simulink model "nmc_full_body_simmechanics_3fbl_2014a"  (R2014a)
settings: Solver=ode23s  StartTime=0.0  StopTime=40  FixedStep=1e-3  MaxStep=ts_max  RelTol=1e-3  AbsTol=1e-4
InitFcn:
  | addpath('../lib');
  | addpath('./init_script');
  | nms_model_MechInit
  | nms_model_ControlInit
undefined symbols (not defined in the file): alphaFmGas, alphaFmGlu, alphaFmHam, alphaFmSol, alphaFmVas, alphaLceHam, alphaLceHfl, alphaLceTa, alphaLceTa1, Amp, amp_var, D12_F, D12_S, D12_T, D13_F, D1G_F, D1G_HAT, D1G_S, D1G_T, freq, freq_var, In_F, In_HAT, In_S, In_T, k_gx, k_gy, k_pressure, m_F, m_HAT, m_S, m_T, mu_slide, mu_stick, sgn, ThPos, v_gx_max, v_gy_max, v_max_pressure, vLimit
libraries: mblibv1 x60, simulink x30, simulink_extras x4, nmc x4
(part 2 of 3)

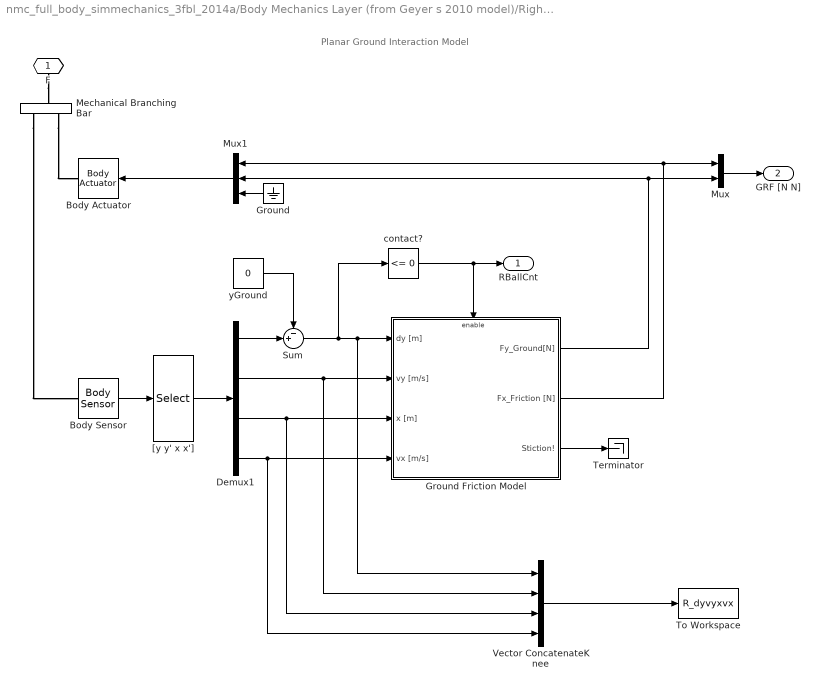
== system nmc_full_body_simmechanics_3fbl_2014a/Body Mechanics Layer (from Geyer s 2010 model)/Right Ball Contact ==
  note: Planar Ground Interaction Model
  Body Actuator : mblibv1/Sensors &  Actuators/Body Actuator  UpdateFromCAD=off  PhysicalDomain=Mechanical  PortType=blob  ActuationStyle=Force  AngleUnits=deg  ArcVelocityUnits=deg/s  ArcAccelerationUnits=deg/s^2  CoordPositionUnits=m  VelocityUnits=m/s  AccelerationUnits=m/s^2  ForceUnits=N  TorqueUnits=N-m  ActiveIO=on  Width=3  DialogClass=MechanicalActuatorBlock  ReferenceFrame=Absolute (World)  Angle=off  CoordPosition=on  Force=on  Torque=off
  Body Sensor : mblibv1/Sensors &  Actuators/Body Sensor  UpdateFromCAD=off  PhysicalDomain=Mechanical  PortType=blob  Muxed=on  Pose=off  Angle=on  AngleUnits=deg  ArcVelocity=off  ArcVelocityUnits=deg/s  ArcAcceleration=off  ArcAccelerationUnits=deg/s^2  CoordPosition=on  CoordPositionUnits=m  Velocity=on  VelocityUnits=m/s  Acceleration=off  AccelerationUnits=m/s^2  Quaternion=on  QuaternionDT=off  QuaternionDDT=off  QuaternionUnits=off  OutputVector=[ 3 3 ]  ActiveIO=on  Width=6  DialogClass=MechanicalSensorBlock  ReferenceFrame=Absolute (World)
  Demux1 : Demux
  Ground : Ground
  Ground Friction Model : Subsystem
  Mechanical Branching Bar : mblibv1/Utilities/Mechanical Branching Bar  LConnTagsString=_newl0  RConnTagsString=SA0|SA1  UpdateFromCAD=off  DialogClass=MechanicalBranchingBarBlock  NumSAPorts=2
  Mux : Mux  Inputs=2
  Mux1 : Mux  Inputs=3
  Sum : Sum  Inputs=-+|
  Terminator : Terminator
  To Workspace : ToWorkspace  VariableName=R_dyvyxvx  SaveFormat=Timeseries  SampleTime=-1
  Vector ConcatenateKnee : Concatenate  NumInputs=4
  "[y y' x x']" : Selector  InputPortWidth=6  IndexOptions=Index vector (dialog)  Indices=[2 5 1 4]  OutputSizes=1
  contact? : simulink/Logic and Bit Operations/Compare To Zero  relop=<=  OutDataTypeStr=boolean
  yGround : Constant  Value=0
  F : PMIOPort  Port=1  Side=Left
  RBallCnt : Outport
  GRF [N N] : Outport  Port=2
  wires:
  Demux1/2 -> Vector ConcatenateKnee/2, Ground Friction Model/2(vy [m/s])
  contact?/1 -> Ground Friction Model/Enable, RBallCnt/1
  Ground Friction Model/1(Fy_Ground[N]) -> Mux/2, Mux1/2
  Ground Friction Model/2(Fx_Friction [N]) -> Mux/1, Mux1/1
  Ground Friction Model/3(Stiction!) -> Terminator/1
  Mux/1 -> GRF [N N]/1
  Sum/1 -> Vector ConcatenateKnee/1, Ground Friction Model/1(dy [m]), contact?/1
  yGround/1 -> Sum/1
  Body Sensor/1 -> "[y y' x x']"/1
  "[y y' x x']"/1 -> Demux1/1
  Demux1/1 -> Sum/2
  Demux1/3 -> Vector ConcatenateKnee/3, Ground Friction Model/3(x [m])
  Demux1/4 -> Vector ConcatenateKnee/4, Ground Friction Model/4(vx [m/s])
  Ground/1 -> Mux1/3
  Mux1/1 -> Body Actuator/1
  Vector ConcatenateKnee/1 -> To Workspace/1
  connections:
  F/RConn1 -- Mechanical Branching Bar/LConn1
  Mechanical Branching Bar/RConn2 -- Body Actuator/RConn1
  Mechanical Branching Bar/RConn1 -- Body Sensor/LConn1

== system nmc_full_body_simmechanics_3fbl_2014a/Body Mechanics Layer (from Geyer s 2010 model)/Right Heel Contact ==
  note: Planar Ground Interaction Model
  Body Actuator : mblibv1/Sensors &  Actuators/Body Actuator  UpdateFromCAD=off  PhysicalDomain=Mechanical  PortType=blob  ActuationStyle=Force  AngleUnits=deg  ArcVelocityUnits=deg/s  ArcAccelerationUnits=deg/s^2  CoordPositionUnits=m  VelocityUnits=m/s  AccelerationUnits=m/s^2  ForceUnits=N  TorqueUnits=N-m  ActiveIO=on  Width=3  DialogClass=MechanicalActuatorBlock  ReferenceFrame=Absolute (World)  Angle=off  CoordPosition=on  Force=on  Torque=off
  Body Sensor : mblibv1/Sensors &  Actuators/Body Sensor  UpdateFromCAD=off  PhysicalDomain=Mechanical  PortType=blob  Muxed=on  Pose=off  Angle=on  AngleUnits=deg  ArcVelocity=off  ArcVelocityUnits=deg/s  ArcAcceleration=off  ArcAccelerationUnits=deg/s^2  CoordPosition=on  CoordPositionUnits=m  Velocity=on  VelocityUnits=m/s  Acceleration=off  AccelerationUnits=m/s^2  Quaternion=on  QuaternionDT=off  QuaternionDDT=off  QuaternionUnits=off  OutputVector=[ 3 3 ]  ActiveIO=on  Width=6  DialogClass=MechanicalSensorBlock  ReferenceFrame=Absolute (World)
  Demux1 : Demux
  Ground : Ground
  Ground Friction Model : Subsystem
  Mechanical Branching Bar : mblibv1/Utilities/Mechanical Branching Bar  LConnTagsString=_newl0  RConnTagsString=SA0|SA1  UpdateFromCAD=off  DialogClass=MechanicalBranchingBarBlock  NumSAPorts=2
  Mux : Mux  Inputs=2
  Mux1 : Mux  Inputs=3
  Sum : Sum  Inputs=-+|
  Terminator : Terminator
  "[y y' x x']" : Selector  InputPortWidth=6  IndexOptions=Index vector (dialog)  Indices=[2 5 1 4]  OutputSizes=1
  contact? : simulink/Logic and Bit Operations/Compare To Zero  relop=<=  OutDataTypeStr=boolean
  yGround : Constant  Value=0
  F : PMIOPort  Port=1  Side=Left
  RHeelCnt : Outport
  GRF [N N] : Outport  Port=2
  wires:
  Ground Friction Model/3(Stiction!) -> Terminator/1
  Ground Friction Model/2(Fx_Friction [N]) -> Mux/1, Mux1/1
  Ground Friction Model/1(Fy_Ground[N]) -> Mux/2, Mux1/2
  contact?/1 -> Ground Friction Model/Enable, RHeelCnt/1
  Demux1/4 -> Ground Friction Model/4(vx [m/s])
  Demux1/3 -> Ground Friction Model/3(x [m])
  Demux1/2 -> Ground Friction Model/2(vy [m/s])
  Mux/1 -> GRF [N N]/1
  yGround/1 -> Sum/1
  Demux1/1 -> Sum/2  "yBall"
  Sum/1 -> Ground Friction Model/1(dy [m]), contact?/1
  Body Sensor/1 -> "[y y' x x']"/1
  "[y y' x x']"/1 -> Demux1/1
  Mux1/1 -> Body Actuator/1
  Ground/1 -> Mux1/3
  connections:
  F/RConn1 -- Mechanical Branching Bar/LConn1
  Mechanical Branching Bar/RConn1 -- Body Sensor/LConn1
  Mechanical Branching Bar/RConn2 -- Body Actuator/RConn1

== system nmc_full_body_simmechanics_3fbl_2014a/Body Mechanics Layer (from Geyer s 2010 model)/Right Force Plate ==
  "GRF_Ball [N N] " : Inport
  GRF_Heel [N N] : Inport  Port=2
  Enable : EnablePort  StatesWhenEnabling=reset
  Fcn : Fcn  Expr=u(1)/(u(2)+eps)
  Mux : Mux  Inputs=3
  Mux1 : Mux  Inputs=2
  Selector : Selector  InputPortWidth=2  IndexOptions=Index vector (dialog)  Indices=2  OutputSizes=1
  Selector1 : Selector  InputPortWidth=2  IndexOptions=Index vector (dialog)  Indices=2  OutputSizes=1
  Sum1 : Sum
  GRFs : Outport  OutputWhenDisabled=reset  InitialOutput=0
  COP : Outport  Port=2  OutputWhenDisabled=reset  InitialOutput=0
  wires:
  Selector/1 -> Mux1/2
  Selector1/1 -> Mux1/1
  "GRF_Ball [N N] "/1 -> Sum1/1, Mux/1, Selector1/1
  GRF_Heel [N N]/1 -> Sum1/2, Mux/3
  Sum1/1 -> Mux/2, Selector/1
  Mux/1 -> GRFs/1
  Mux1/1 -> Fcn/1
  Fcn/1 -> COP/1

== system nmc_full_body_simmechanics_3fbl_2014a/Body Mechanics Layer (from Geyer s 2010 model)/Right Thigh Sensor Sheet ==
  note: Inner Segment Pressure Sheet
  Gain3 : Gain  Gain=k_pressure
  Gain4 : Gain  Gain=1/v_max_pressure
  Inner Thigh Shift Joint : mblibv1/Joints/Prismatic  LConnTagsString=__newl0|SA1|SA2  RConnTagsString=__newr0|SA1  UpdateFromCAD=off  NumSAPorts=3  CutJoint=off  MarkAsCut=off  Primitives=prismatic  PrimitiveProps=P1$WORLD$[1 0 0]$prismatic  DialogClass=JointBlock  P1Axis=[1 0 0]
  Mux1 : Mux  Inputs=2
  Pressure Sheet Reaction Force : Fcn  Expr=-u(1) * (1+sgn(u(1))*u(2))
  Right Thigh Sensor Sheet IC : mblibv1/Sensors &  Actuators/Joint Initial Condition  UpdateFromCAD=off  LeftPortType=blob  RightPortType=blob  PhysicalDomain=mechanical  DialogClass=InitialConditionBlock  InitialConditions=P1$true$0$m$rad$0$m/s$rad/s#P2$false$0$m$rad$0$m/s$rad/s#P3$false$0$m$rad$0$m/s$rad/s#R1$false$0$m$rad$0$m/s$rad/s#R2$false$0$m$rad$0$m/s$rad/s#R3$false$0$m$rad$0$m/s$rad/s#S$false$0$m$rad$0$m/s$rad/s  P1PIC=0  P1VIC=0  P2PIC=0  P2VIC=0  P3PIC=0  P3VIC=0  R1PIC=0  R1VIC=0  R2PIC=0  R2VIC=0  R3PIC=0  R3VIC=0  SPIC=0  SVIC=0
  Thigh Actuator : mblibv1/Sensors &  Actuators/Joint Actuator  UpdateFromCAD=off  PhysicalDomain=Mechanical  PortType=blob  ActuationStyle=Force  AngleUnits=deg  ArcVelocityUnits=deg/s  ArcAccelerationUnits=deg/s^2  CoordPositionUnits=m  VelocityUnits=m/s  AccelerationUnits=m/s^2  ForceUnits=N  TorqueUnits=N-m  ActiveIO=on  Width=1  DialogClass=MechanicalActuatorBlock  Primitive=P1  ReferenceFrame=Absolute (INERTIAL)
  Thigh Sensor : mblibv1/Sensors &  Actuators/Joint Sensor  UpdateFromCAD=off  PhysicalDomain=Mechanical  PortType=blob  Muxed=off  Pose=off  Angle=on  AngleUnits=deg  ArcVelocity=off  ArcVelocityUnits=deg/s  ArcAcceleration=off  ArcAccelerationUnits=deg/s^2  CoordPosition=on  CoordPositionUnits=m  Velocity=on  VelocityUnits=m/s  Acceleration=off  AccelerationUnits=m/s^2  Quaternion=on  QuaternionDT=off  QuaternionDDT=off  QuaternionUnits=off  OutputVector=[ 1 1 ]  ActiveIO=on  Width=2  DialogClass=MechanicalSensorBlock  Primitive=P1  Force=off  ForceUnits=N  Torque=off  TorqueUnits=N-m  ReferenceFrame=Absolute (INERTIAL)  ReactionSensedSide=Base  ReactionReferenceFrame=Absolute (World)  ReactionForce=off  ReactionForceUnits=N  ReactionMoment=off  ReactionMomentUnits=N-m
  B : PMIOPort  Tag=PMCPort  Port=1  Side=Left
  F : PMIOPort  Tag=PMCPort  Port=2  Side=Right
  dx : Outport
  wires:
  Thigh Sensor/1 -> Gain3/1, dx/1
  Thigh Sensor/2 -> Gain4/1
  Mux1/1 -> Pressure Sheet Reaction Force/1
  Gain3/1 -> Mux1/1
  Gain4/1 -> Mux1/2
  Pressure Sheet Reaction Force/1 -> Thigh Actuator/1
  connections:
  B/RConn1 -- Inner Thigh Shift Joint/LConn1
  F/RConn1 -- Inner Thigh Shift Joint/RConn1
  Thigh Sensor/LConn1 -- Inner Thigh Shift Joint/LConn2
  Inner Thigh Shift Joint/RConn2 -- Thigh Actuator/RConn1
  Inner Thigh Shift Joint/LConn3 -- Right Thigh Sensor Sheet IC/RConn1

== system nmc_full_body_simmechanics_3fbl_2014a/Full Body Control (created using the nmc library)/Subsystem ==
  Parameter variation : Subsystem

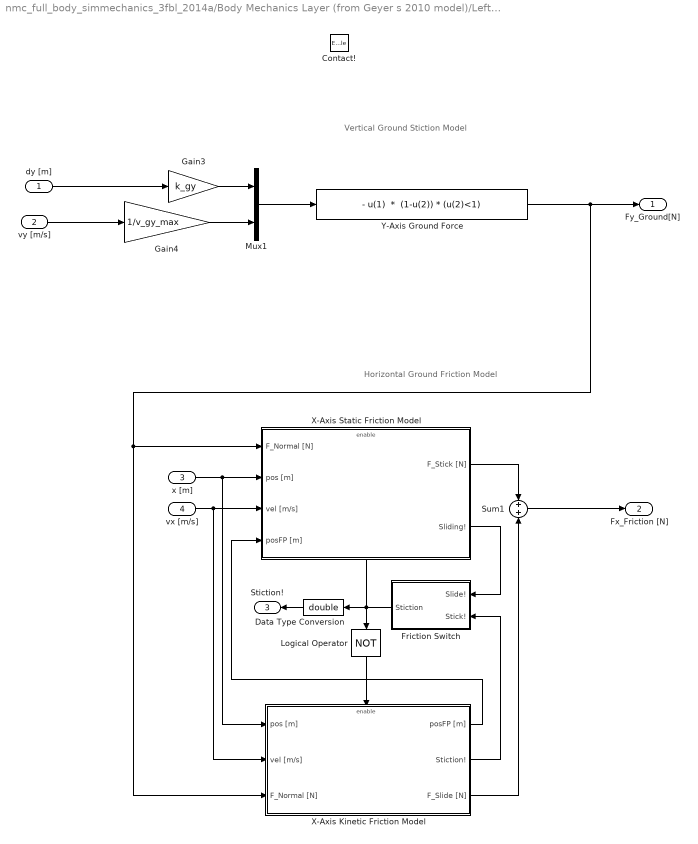
== system nmc_full_body_simmechanics_3fbl_2014a/Body Mechanics Layer (from Geyer s 2010 model)/Left Ball Contact/Ground Friction Model ==
  note: Horizontal Ground Friction Model
  note: Vertical Ground Stiction Model
  dy [m] : Inport
  vy [m/s] : Inport  Port=2
  x [m] : Inport  Port=3
  vx [m/s] : Inport  Port=4
  Contact! : EnablePort  StatesWhenEnabling=reset
  Data Type Conversion : DataTypeConversion  OutDataTypeStr=double
  Friction Switch : Subsystem
  Gain3 : Gain  Gain=k_gy
  Gain4 : Gain  Gain=1/v_gy_max
  Logical Operator : Logic  Operator=NOT  AllPortsSameDT=off  OutDataTypeStr=boolean
  Mux1 : Mux  Inputs=2
  Sum1 : Sum
  X-Axis Kinetic Friction Model : Subsystem
  X-Axis Static Friction Model : Subsystem
  Y-Axis Ground Force : Fcn  Expr="- u(1)  *  (1-u(2)) * (u(2)<1)"
  Fy_Ground[N] : Outport  OutputWhenDisabled=reset  InitialOutput=0
      settings: AttributesFormatString=initial = '%<InitialOutput>'\nwhen disabled = '%<OutputWhenDisabled>'
  Fx_Friction [N] : Outport  Port=2  OutputWhenDisabled=reset  InitialOutput=0
      settings: AttributesFormatString=initial = '%<InitialOutput>'\nwhen\ndisabled\n'%<OutputWhenDisabled>'
  Stiction! : Outport  Port=3  OutputWhenDisabled=reset  InitialOutput=0
      settings: AttributesFormatString=initial = '%<InitialOutput>'\nwhen\ndisabled\n'%<OutputWhenDisabled>'
  wires:
  dy [m]/1 -> Gain3/1
  vy [m/s]/1 -> Gain4/1
  x [m]/1 -> X-Axis Static Friction Model/2(pos [m]), X-Axis Kinetic Friction Model/1(pos [m])
  vx [m/s]/1 -> X-Axis Static Friction Model/3(vel [m/s]), X-Axis Kinetic Friction Model/2(vel [m/s])
  X-Axis Kinetic Friction Model/1(posFP [m]) -> X-Axis Static Friction Model/4(posFP [m])
  X-Axis Kinetic Friction Model/3(F_Slide [N]) -> Sum1/2
  X-Axis Static Friction Model/1(F_Stick [N]) -> Sum1/1
  Sum1/1 -> Fx_Friction [N]/1
  Friction Switch/1(Stiction) -> X-Axis Static Friction Model/Enable, Logical Operator/1, Data Type Conversion/1
  X-Axis Static Friction Model/2(Sliding!) -> Friction Switch/1(Slide!)
  X-Axis Kinetic Friction Model/2(Stiction!) -> Friction Switch/2(Stick!)
  Logical Operator/1 -> X-Axis Kinetic Friction Model/Enable
  Data Type Conversion/1 -> Stiction!/1
  Mux1/1 -> Y-Axis Ground Force/1
  Gain3/1 -> Mux1/1
  Gain4/1 -> Mux1/2
  Y-Axis Ground Force/1 -> Fy_Ground[N]/1, X-Axis Static Friction Model/1(F_Normal [N]), X-Axis Kinetic Friction Model/3(F_Normal [N])

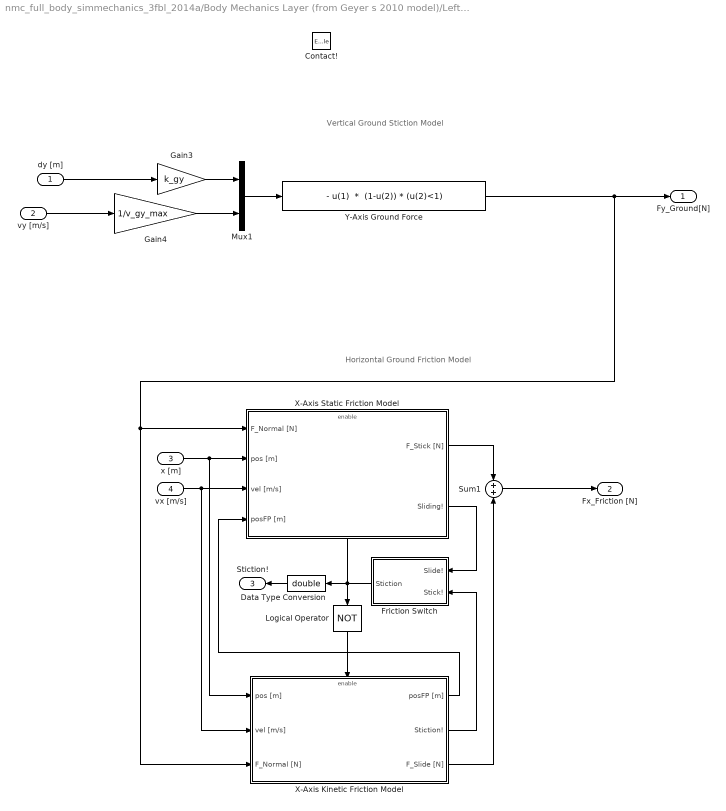
== system nmc_full_body_simmechanics_3fbl_2014a/Body Mechanics Layer (from Geyer s 2010 model)/Left Heel Contact/Ground Friction Model ==
  note: Vertical Ground Stiction Model
  note: Horizontal Ground Friction Model
  dy [m] : Inport
  vy [m/s] : Inport  Port=2
  x [m] : Inport  Port=3
  vx [m/s] : Inport  Port=4
  Contact! : EnablePort  StatesWhenEnabling=reset
  Data Type Conversion : DataTypeConversion  OutDataTypeStr=double
  Friction Switch : Subsystem
  Gain3 : Gain  Gain=k_gy
  Gain4 : Gain  Gain=1/v_gy_max
  Logical Operator : Logic  Operator=NOT  AllPortsSameDT=off  OutDataTypeStr=boolean
  Mux1 : Mux  Inputs=2
  Sum1 : Sum
  X-Axis Kinetic Friction Model : Subsystem
  X-Axis Static Friction Model : Subsystem
  Y-Axis Ground Force : Fcn  Expr="- u(1)  *  (1-u(2)) * (u(2)<1)"
  Fy_Ground[N] : Outport  OutputWhenDisabled=reset  InitialOutput=0
      settings: AttributesFormatString=initial = '%<InitialOutput>'\nwhen disabled = '%<OutputWhenDisabled>'
  Fx_Friction [N] : Outport  Port=2  OutputWhenDisabled=reset  InitialOutput=0
      settings: AttributesFormatString=initial = '%<InitialOutput>'\nwhen\ndisabled\n'%<OutputWhenDisabled>'
  Stiction! : Outport  Port=3  OutputWhenDisabled=reset  InitialOutput=0
      settings: AttributesFormatString=initial = '%<InitialOutput>'\nwhen\ndisabled\n'%<OutputWhenDisabled>'
  wires:
  Gain4/1 -> Mux1/2
  Gain3/1 -> Mux1/1
  Mux1/1 -> Y-Axis Ground Force/1
  Data Type Conversion/1 -> Stiction!/1
  Logical Operator/1 -> X-Axis Kinetic Friction Model/Enable
  X-Axis Kinetic Friction Model/2(Stiction!) -> Friction Switch/2(Stick!)
  X-Axis Static Friction Model/2(Sliding!) -> Friction Switch/1(Slide!)
  Friction Switch/1(Stiction) -> Data Type Conversion/1, Logical Operator/1, X-Axis Static Friction Model/Enable
  Sum1/1 -> Fx_Friction [N]/1
  X-Axis Static Friction Model/1(F_Stick [N]) -> Sum1/1
  X-Axis Kinetic Friction Model/3(F_Slide [N]) -> Sum1/2
  X-Axis Kinetic Friction Model/1(posFP [m]) -> X-Axis Static Friction Model/4(posFP [m])
  vx [m/s]/1 -> X-Axis Kinetic Friction Model/2(vel [m/s]), X-Axis Static Friction Model/3(vel [m/s])
  x [m]/1 -> X-Axis Kinetic Friction Model/1(pos [m]), X-Axis Static Friction Model/2(pos [m])
  vy [m/s]/1 -> Gain4/1
  dy [m]/1 -> Gain3/1
  Y-Axis Ground Force/1 -> Fy_Ground[N]/1, X-Axis Kinetic Friction Model/3(F_Normal [N]), X-Axis Static Friction Model/1(F_Normal [N])

== system nmc_full_body_simmechanics_3fbl_2014a/Body Mechanics Layer (from Geyer s 2010 model)/Right Ball Contact/Ground Friction Model ==
  note: Horizontal Ground Friction Model
  note: Vertical Ground Stiction Model
  dy [m] : Inport
  vy [m/s] : Inport  Port=2
  x [m] : Inport  Port=3
  vx [m/s] : Inport  Port=4
  Contact! : EnablePort  StatesWhenEnabling=reset
  Data Type Conversion : DataTypeConversion  OutDataTypeStr=double
  Friction Switch : Subsystem
  Gain3 : Gain  Gain=k_gy
  Gain4 : Gain  Gain=1/v_gy_max
  Logical Operator : Logic  Operator=NOT  AllPortsSameDT=off  OutDataTypeStr=boolean
  Mux1 : Mux  Inputs=2
  Sum1 : Sum
  X-Axis Kinetic Friction Model : Subsystem
  X-Axis Static Friction Model : Subsystem
  Y-Axis Ground Force : Fcn  Expr="- u(1)  *  (1-u(2)) * (u(2)<1)"
  Fy_Ground[N] : Outport  OutputWhenDisabled=reset  InitialOutput=0
      settings: AttributesFormatString=initial = '%<InitialOutput>'\nwhen disabled = '%<OutputWhenDisabled>'
  Fx_Friction [N] : Outport  Port=2  OutputWhenDisabled=reset  InitialOutput=0
      settings: AttributesFormatString=initial = '%<InitialOutput>'\nwhen\ndisabled\n'%<OutputWhenDisabled>'
  Stiction! : Outport  Port=3  OutputWhenDisabled=reset  InitialOutput=0
      settings: AttributesFormatString=initial = '%<InitialOutput>'\nwhen\ndisabled\n'%<OutputWhenDisabled>'
  wires:
  dy [m]/1 -> Gain3/1
  vy [m/s]/1 -> Gain4/1
  x [m]/1 -> X-Axis Static Friction Model/2(pos [m]), X-Axis Kinetic Friction Model/1(pos [m])
  vx [m/s]/1 -> X-Axis Static Friction Model/3(vel [m/s]), X-Axis Kinetic Friction Model/2(vel [m/s])
  X-Axis Kinetic Friction Model/1(posFP [m]) -> X-Axis Static Friction Model/4(posFP [m])
  X-Axis Kinetic Friction Model/3(F_Slide [N]) -> Sum1/2
  X-Axis Static Friction Model/1(F_Stick [N]) -> Sum1/1
  Sum1/1 -> Fx_Friction [N]/1
  Friction Switch/1(Stiction) -> X-Axis Static Friction Model/Enable, Logical Operator/1, Data Type Conversion/1
  X-Axis Static Friction Model/2(Sliding!) -> Friction Switch/1(Slide!)
  X-Axis Kinetic Friction Model/2(Stiction!) -> Friction Switch/2(Stick!)
  Logical Operator/1 -> X-Axis Kinetic Friction Model/Enable
  Data Type Conversion/1 -> Stiction!/1
  Mux1/1 -> Y-Axis Ground Force/1
  Gain3/1 -> Mux1/1
  Gain4/1 -> Mux1/2
  Y-Axis Ground Force/1 -> Fy_Ground[N]/1, X-Axis Static Friction Model/1(F_Normal [N]), X-Axis Kinetic Friction Model/3(F_Normal [N])

== system nmc_full_body_simmechanics_3fbl_2014a/Body Mechanics Layer (from Geyer s 2010 model)/Right Heel Contact/Ground Friction Model ==
  note: Vertical Ground Stiction Model
  note: Horizontal Ground Friction Model
  dy [m] : Inport
  vy [m/s] : Inport  Port=2
  x [m] : Inport  Port=3
  vx [m/s] : Inport  Port=4
  Contact! : EnablePort  StatesWhenEnabling=reset
  Data Type Conversion : DataTypeConversion  OutDataTypeStr=double
  Friction Switch : Subsystem
  Gain3 : Gain  Gain=k_gy
  Gain4 : Gain  Gain=1/v_gy_max
  Logical Operator : Logic  Operator=NOT  AllPortsSameDT=off  OutDataTypeStr=boolean
  Mux1 : Mux  Inputs=2
  Sum1 : Sum
  X-Axis Kinetic Friction Model : Subsystem
  X-Axis Static Friction Model : Subsystem
  Y-Axis Ground Force : Fcn  Expr="- u(1)  *  (1-u(2)) * (u(2)<1)"
  Fy_Ground[N] : Outport  OutputWhenDisabled=reset  InitialOutput=0
      settings: AttributesFormatString=initial = '%<InitialOutput>'\nwhen disabled = '%<OutputWhenDisabled>'
  Fx_Friction [N] : Outport  Port=2  OutputWhenDisabled=reset  InitialOutput=0
      settings: AttributesFormatString=initial = '%<InitialOutput>'\nwhen\ndisabled\n'%<OutputWhenDisabled>'
  Stiction! : Outport  Port=3  OutputWhenDisabled=reset  InitialOutput=0
      settings: AttributesFormatString=initial = '%<InitialOutput>'\nwhen\ndisabled\n'%<OutputWhenDisabled>'
  wires:
  Gain4/1 -> Mux1/2
  Gain3/1 -> Mux1/1
  Mux1/1 -> Y-Axis Ground Force/1
  Data Type Conversion/1 -> Stiction!/1
  Logical Operator/1 -> X-Axis Kinetic Friction Model/Enable
  X-Axis Kinetic Friction Model/2(Stiction!) -> Friction Switch/2(Stick!)
  X-Axis Static Friction Model/2(Sliding!) -> Friction Switch/1(Slide!)
  Friction Switch/1(Stiction) -> Data Type Conversion/1, Logical Operator/1, X-Axis Static Friction Model/Enable
  Sum1/1 -> Fx_Friction [N]/1
  X-Axis Static Friction Model/1(F_Stick [N]) -> Sum1/1
  X-Axis Kinetic Friction Model/3(F_Slide [N]) -> Sum1/2
  X-Axis Kinetic Friction Model/1(posFP [m]) -> X-Axis Static Friction Model/4(posFP [m])
  vx [m/s]/1 -> X-Axis Kinetic Friction Model/2(vel [m/s]), X-Axis Static Friction Model/3(vel [m/s])
  x [m]/1 -> X-Axis Kinetic Friction Model/1(pos [m]), X-Axis Static Friction Model/2(pos [m])
  vy [m/s]/1 -> Gain4/1
  dy [m]/1 -> Gain3/1
  Y-Axis Ground Force/1 -> Fy_Ground[N]/1, X-Axis Kinetic Friction Model/3(F_Normal [N]), X-Axis Static Friction Model/1(F_Normal [N])

== system nmc_full_body_simmechanics_3fbl_2014a/Full Body Control (created using the nmc library)/Subsystem/Parameter variation ==
  Alpha variation : Subsystem  Commented=on
  Amplitude Variation : Subsystem  Commented=on
  Freq variation : Subsystem  Commented=on

== system nmc_full_body_simmechanics_3fbl_2014a/Body Mechanics Layer (from Geyer s 2010 model)/Left Ball Contact/Ground Friction Model/Friction Switch ==
  note: Static/Kinetic Friction Switch
  Slide! : Inport
  Stick! : Inport  Port=2
  Memory : Memory
  S-R Flip-Flop : simulink_extras/Flip Flops/S-R Flip-Flop  initial_condition=1
  Terminator : Terminator
  Stiction : Outport
  wires:
  S-R Flip-Flop/1 -> Memory/1
  S-R Flip-Flop/2 -> Terminator/1
  Stick!/1 -> S-R Flip-Flop/1
  Slide!/1 -> S-R Flip-Flop/2
  Memory/1 -> Stiction/1

== system nmc_full_body_simmechanics_3fbl_2014a/Body Mechanics Layer (from Geyer s 2010 model)/Left Ball Contact/Ground Friction Model/X-Axis Kinetic Friction Model ==
  note: Kinetic Friction Model
  note: Footpoint Determiner
  note: Sliding Limit Detector
  pos [m] : Inport
  vel [m/s] : Inport  Port=2
  F_Normal [N] : Inport  Port=3
  Enable : EnablePort  StatesWhenEnabling=reset  ZeroCross=off
  Abs : Abs
  Constant : Constant  Value=vLimit
  FixPt Relational Operator : RelationalOperator  Operator=>  OutDataTypeStr=boolean  ZeroCross=off
  Memory : Memory
  Negative : simulink/Logic and Bit Operations/Compare To Zero  relop=<  OutDataTypeStr=boolean
  Product : Product  RndMeth=Zero
  Sign1 : Signum
  Sum : Sum  Inputs=|+-
  reverse : Gain  Gain=-1
  sliding friction coefficient : Gain  Gain=mu_slide
  posFP [m] : Outport  InitialOutput=0
      settings: AttributesFormatString=initial = '%<InitialOutput>'\nwhen disabled = '%<OutputWhenDisabled>'
  Stiction! : Outport  Port=2  OutputWhenDisabled=reset  InitialOutput=0
      settings: AttributesFormatString=initial = '%<InitialOutput>'\nwhen disabled = '%<OutputWhenDisabled>'
  F_Slide [N] : Outport  Port=3  OutputWhenDisabled=reset  InitialOutput=0
      settings: AttributesFormatString=initial = '%<InitialOutput>'\nwhen disabled = '%<OutputWhenDisabled>'
  wires:
  reverse/1 -> Product/1
  F_Normal [N]/1 -> sliding friction coefficient/1
  vel [m/s]/1 -> Sign1/1, Abs/1
  pos [m]/1 -> posFP [m]/1
  Product/1 -> F_Slide [N]/1
  sliding friction coefficient/1 -> Product/2
  Sign1/1 -> reverse/1
  FixPt Relational Operator/1 -> Stiction!/1
  Memory/1 -> FixPt Relational Operator/2
  Negative/1 -> FixPt Relational Operator/1, Memory/1
  Abs/1 -> Sum/1
  Sum/1 -> Negative/1
  Constant/1 -> Sum/2

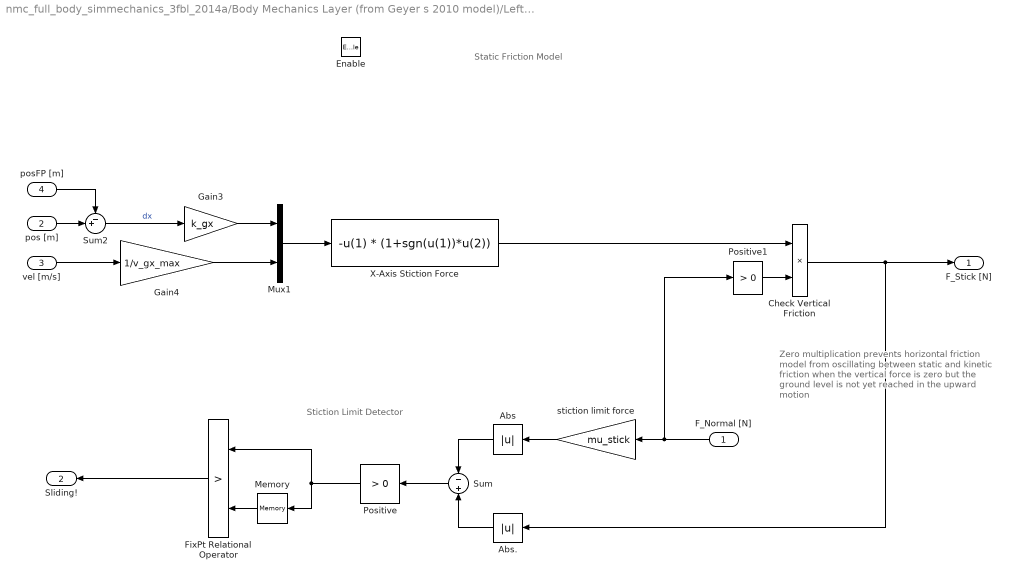
== system nmc_full_body_simmechanics_3fbl_2014a/Body Mechanics Layer (from Geyer s 2010 model)/Left Ball Contact/Ground Friction Model/X-Axis Static Friction Model ==
  note: Stiction Limit Detector
  note: Static Friction Model
  note: Zero multiplication prevents
      | horizontal friction model from
      | oscillating between static and kinetic
      | friction when the vertical force is zero but
      | the ground level is not yet reached
      | in the upward motion
  F_Normal [N] : Inport
  pos [m] : Inport  Port=2
  vel [m/s] : Inport  Port=3
  posFP [m] : Inport  Port=4
  Enable : EnablePort  StatesWhenEnabling=reset  ZeroCross=off
  Abs : Abs
  Abs. : Abs
  Check Vertical Friction : Product  RndMeth=Zero
  FixPt Relational Operator : RelationalOperator  Operator=>  OutDataTypeStr=boolean  ZeroCross=off
  Gain3 : Gain  Gain=k_gx
  Gain4 : Gain  Gain=1/v_gx_max
  Memory : Memory
  Mux1 : Mux  Inputs=2
  Positive : simulink/Logic and Bit Operations/Compare To Zero  relop=>  OutDataTypeStr=boolean
  Positive1 : simulink/Logic and Bit Operations/Compare To Zero  relop=>  OutDataTypeStr=boolean
  Sum : Sum  Inputs=-+
  Sum2 : Sum  Inputs=-+|
  X-Axis Stiction Force : Fcn  Expr=-u(1) * (1+sgn(u(1))*u(2))
  stiction limit force : Gain  Gain=mu_stick
  F_Stick [N] : Outport  OutputWhenDisabled=reset  InitialOutput=0
      settings: AttributesFormatString=when disabled: %<OutputWhenDisabled>\ninitial: %<InitialOutput>
  Sliding! : Outport  Port=2  OutputWhenDisabled=reset  InitialOutput=0
      settings: AttributesFormatString=when disabled: %<OutputWhenDisabled>\ninitial: %<InitialOutput>
  wires:
  F_Normal [N]/1 -> stiction limit force/1, Positive1/1
  Sum2/1 -> Gain3/1  "dx"
  pos [m]/1 -> Sum2/2
  posFP [m]/1 -> Sum2/1
  vel [m/s]/1 -> Gain4/1
  Sum/1 -> Positive/1
  Memory/1 -> FixPt Relational Operator/2
  Positive/1 -> FixPt Relational Operator/1, Memory/1
  Abs./1 -> Sum/2
  Mux1/1 -> X-Axis Stiction Force/1
  Gain3/1 -> Mux1/1
  Gain4/1 -> Mux1/2
  FixPt Relational Operator/1 -> Sliding!/1
  Abs/1 -> Sum/1
  stiction limit force/1 -> Abs/1
  X-Axis Stiction Force/1 -> Check Vertical Friction/1
  Positive1/1 -> Check Vertical Friction/2
  Check Vertical Friction/1 -> F_Stick [N]/1, Abs./1

== system nmc_full_body_simmechanics_3fbl_2014a/Body Mechanics Layer (from Geyer s 2010 model)/Left Heel Contact/Ground Friction Model/Friction Switch ==
  note: Static/Kinetic Friction Switch
  Slide! : Inport
  Stick! : Inport  Port=2
  Memory : Memory
  S-R Flip-Flop : simulink_extras/Flip Flops/S-R Flip-Flop  initial_condition=1
  Terminator : Terminator
  Stiction : Outport
  wires:
  Memory/1 -> Stiction/1
  Slide!/1 -> S-R Flip-Flop/2
  Stick!/1 -> S-R Flip-Flop/1
  S-R Flip-Flop/2 -> Terminator/1
  S-R Flip-Flop/1 -> Memory/1

== system nmc_full_body_simmechanics_3fbl_2014a/Body Mechanics Layer (from Geyer s 2010 model)/Left Heel Contact/Ground Friction Model/X-Axis Kinetic Friction Model ==
  note: Sliding Limit Detector
  note: Footpoint Determiner
  note: Kinetic Friction Model
  pos [m] : Inport
  vel [m/s] : Inport  Port=2
  F_Normal [N] : Inport  Port=3
  Enable : EnablePort  StatesWhenEnabling=reset  ZeroCross=off
  Abs : Abs
  Constant : Constant  Value=vLimit
  FixPt Relational Operator : RelationalOperator  Operator=>  OutDataTypeStr=boolean  ZeroCross=off
  Memory : Memory
  Negative : simulink/Logic and Bit Operations/Compare To Zero  relop=<  OutDataTypeStr=boolean
  Product : Product  RndMeth=Zero
  Sign1 : Signum
  Sum : Sum  Inputs=|+-
  reverse : Gain  Gain=-1
  sliding friction coefficient : Gain  Gain=mu_slide
  posFP [m] : Outport  InitialOutput=0
      settings: AttributesFormatString=initial = '%<InitialOutput>'\nwhen disabled = '%<OutputWhenDisabled>'
  Stiction! : Outport  Port=2  OutputWhenDisabled=reset  InitialOutput=0
      settings: AttributesFormatString=initial = '%<InitialOutput>'\nwhen disabled = '%<OutputWhenDisabled>'
  F_Slide [N] : Outport  Port=3  OutputWhenDisabled=reset  InitialOutput=0
      settings: AttributesFormatString=initial = '%<InitialOutput>'\nwhen disabled = '%<OutputWhenDisabled>'
  wires:
  Constant/1 -> Sum/2
  Sum/1 -> Negative/1
  Abs/1 -> Sum/1
  Negative/1 -> Memory/1, FixPt Relational Operator/1
  Memory/1 -> FixPt Relational Operator/2
  FixPt Relational Operator/1 -> Stiction!/1
  Sign1/1 -> reverse/1
  sliding friction coefficient/1 -> Product/2
  Product/1 -> F_Slide [N]/1
  pos [m]/1 -> posFP [m]/1
  vel [m/s]/1 -> Abs/1, Sign1/1
  F_Normal [N]/1 -> sliding friction coefficient/1
  reverse/1 -> Product/1

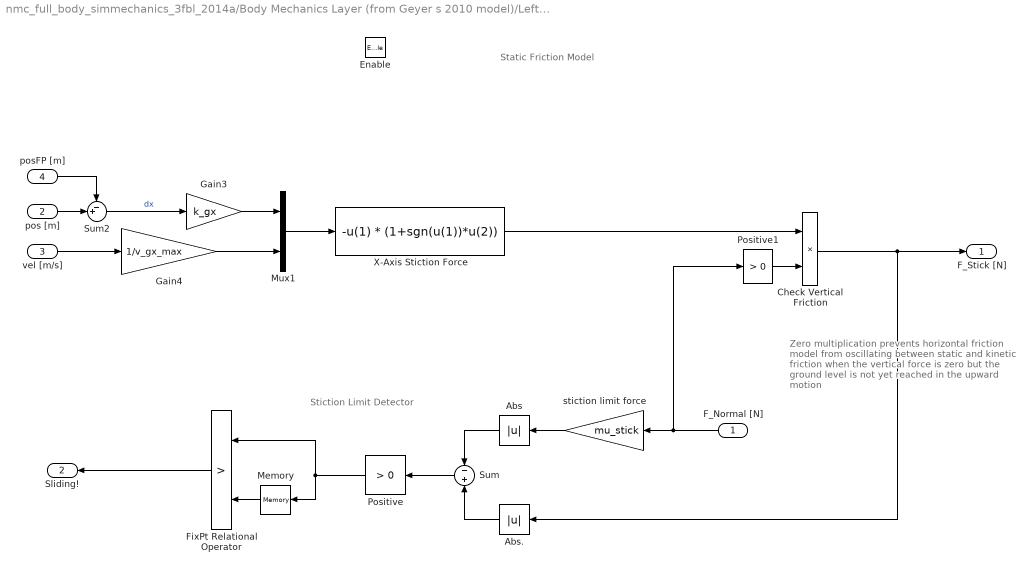
== system nmc_full_body_simmechanics_3fbl_2014a/Body Mechanics Layer (from Geyer s 2010 model)/Left Heel Contact/Ground Friction Model/X-Axis Static Friction Model ==
  note: Static Friction Model
  note: Stiction Limit Detector
  note: Zero multiplication prevents
      | horizontal friction model from
      | oscillating between static and kinetic
      | friction when the vertical force is zero but
      | the ground level is not yet reached
      | in the upward motion
  F_Normal [N] : Inport
  pos [m] : Inport  Port=2
  vel [m/s] : Inport  Port=3
  posFP [m] : Inport  Port=4
  Enable : EnablePort  StatesWhenEnabling=reset  ZeroCross=off
  Abs : Abs
  Abs. : Abs
  Check Vertical Friction : Product  RndMeth=Zero
  FixPt Relational Operator : RelationalOperator  Operator=>  OutDataTypeStr=boolean  ZeroCross=off
  Gain3 : Gain  Gain=k_gx
  Gain4 : Gain  Gain=1/v_gx_max
  Memory : Memory
  Mux1 : Mux  Inputs=2
  Positive : simulink/Logic and Bit Operations/Compare To Zero  relop=>  OutDataTypeStr=boolean
  Positive1 : simulink/Logic and Bit Operations/Compare To Zero  relop=>  OutDataTypeStr=boolean
  Sum : Sum  Inputs=-+
  Sum2 : Sum  Inputs=-+|
  X-Axis Stiction Force : Fcn  Expr=-u(1) * (1+sgn(u(1))*u(2))
  stiction limit force : Gain  Gain=mu_stick
  F_Stick [N] : Outport  OutputWhenDisabled=reset  InitialOutput=0
      settings: AttributesFormatString=when disabled: %<OutputWhenDisabled>\ninitial: %<InitialOutput>
  Sliding! : Outport  Port=2  OutputWhenDisabled=reset  InitialOutput=0
      settings: AttributesFormatString=when disabled: %<OutputWhenDisabled>\ninitial: %<InitialOutput>
  wires:
  F_Normal [N]/1 -> stiction limit force/1, Positive1/1
  Sum2/1 -> Gain3/1  "dx"
  pos [m]/1 -> Sum2/2
  posFP [m]/1 -> Sum2/1
  vel [m/s]/1 -> Gain4/1
  Sum/1 -> Positive/1
  Memory/1 -> FixPt Relational Operator/2
  Positive/1 -> FixPt Relational Operator/1, Memory/1
  Abs./1 -> Sum/2
  Mux1/1 -> X-Axis Stiction Force/1
  Gain3/1 -> Mux1/1
  Gain4/1 -> Mux1/2
  FixPt Relational Operator/1 -> Sliding!/1
  Abs/1 -> Sum/1
  stiction limit force/1 -> Abs/1
  X-Axis Stiction Force/1 -> Check Vertical Friction/1
  Positive1/1 -> Check Vertical Friction/2
  Check Vertical Friction/1 -> F_Stick [N]/1, Abs./1

== system nmc_full_body_simmechanics_3fbl_2014a/Body Mechanics Layer (from Geyer s 2010 model)/Right Ball Contact/Ground Friction Model/Friction Switch ==
  note: Static/Kinetic Friction Switch
  Slide! : Inport
  Stick! : Inport  Port=2
  Memory : Memory
  S-R Flip-Flop : simulink_extras/Flip Flops/S-R Flip-Flop  initial_condition=1
  Terminator : Terminator
  Stiction : Outport
  wires:
  S-R Flip-Flop/1 -> Memory/1
  S-R Flip-Flop/2 -> Terminator/1
  Stick!/1 -> S-R Flip-Flop/1
  Slide!/1 -> S-R Flip-Flop/2
  Memory/1 -> Stiction/1

== system nmc_full_body_simmechanics_3fbl_2014a/Body Mechanics Layer (from Geyer s 2010 model)/Right Ball Contact/Ground Friction Model/X-Axis Kinetic Friction Model ==
  note: Kinetic Friction Model
  note: Footpoint Determiner
  note: Sliding Limit Detector
  pos [m] : Inport
  vel [m/s] : Inport  Port=2
  F_Normal [N] : Inport  Port=3
  Enable : EnablePort  StatesWhenEnabling=reset  ZeroCross=off
  Abs : Abs
  Constant : Constant  Value=vLimit
  FixPt Relational Operator : RelationalOperator  Operator=>  OutDataTypeStr=boolean  ZeroCross=off
  Memory : Memory
  Negative : simulink/Logic and Bit Operations/Compare To Zero  relop=<  OutDataTypeStr=boolean
  Product : Product  RndMeth=Zero
  Sign1 : Signum
  Sum : Sum  Inputs=|+-
  reverse : Gain  Gain=-1
  sliding friction coefficient : Gain  Gain=mu_slide
  posFP [m] : Outport  InitialOutput=0
      settings: AttributesFormatString=initial = '%<InitialOutput>'\nwhen disabled = '%<OutputWhenDisabled>'
  Stiction! : Outport  Port=2  OutputWhenDisabled=reset  InitialOutput=0
      settings: AttributesFormatString=initial = '%<InitialOutput>'\nwhen disabled = '%<OutputWhenDisabled>'
  F_Slide [N] : Outport  Port=3  OutputWhenDisabled=reset  InitialOutput=0
      settings: AttributesFormatString=initial = '%<InitialOutput>'\nwhen disabled = '%<OutputWhenDisabled>'
  wires:
  reverse/1 -> Product/1
  F_Normal [N]/1 -> sliding friction coefficient/1
  vel [m/s]/1 -> Sign1/1, Abs/1
  pos [m]/1 -> posFP [m]/1
  Product/1 -> F_Slide [N]/1
  sliding friction coefficient/1 -> Product/2
  Sign1/1 -> reverse/1
  FixPt Relational Operator/1 -> Stiction!/1
  Memory/1 -> FixPt Relational Operator/2
  Negative/1 -> FixPt Relational Operator/1, Memory/1
  Abs/1 -> Sum/1
  Sum/1 -> Negative/1
  Constant/1 -> Sum/2

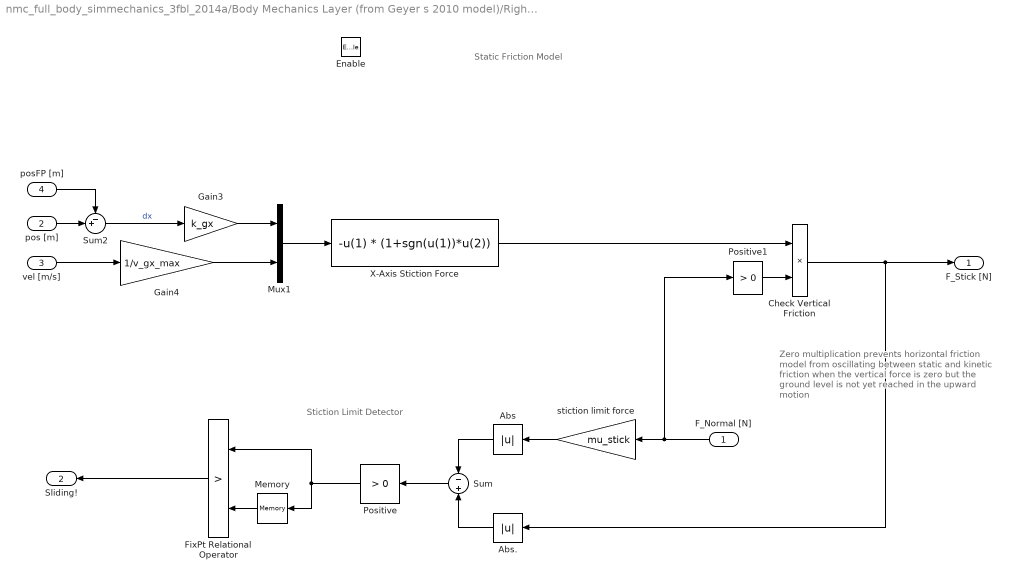
== system nmc_full_body_simmechanics_3fbl_2014a/Body Mechanics Layer (from Geyer s 2010 model)/Right Ball Contact/Ground Friction Model/X-Axis Static Friction Model ==
  note: Stiction Limit Detector
  note: Static Friction Model
  note: Zero multiplication prevents
      | horizontal friction model from
      | oscillating between static and kinetic
      | friction when the vertical force is zero but
      | the ground level is not yet reached
      | in the upward motion
  F_Normal [N] : Inport
  pos [m] : Inport  Port=2
  vel [m/s] : Inport  Port=3
  posFP [m] : Inport  Port=4
  Enable : EnablePort  StatesWhenEnabling=reset  ZeroCross=off
  Abs : Abs
  Abs. : Abs
  Check Vertical Friction : Product  RndMeth=Zero
  FixPt Relational Operator : RelationalOperator  Operator=>  OutDataTypeStr=boolean  ZeroCross=off
  Gain3 : Gain  Gain=k_gx
  Gain4 : Gain  Gain=1/v_gx_max
  Memory : Memory
  Mux1 : Mux  Inputs=2
  Positive : simulink/Logic and Bit Operations/Compare To Zero  relop=>  OutDataTypeStr=boolean
  Positive1 : simulink/Logic and Bit Operations/Compare To Zero  relop=>  OutDataTypeStr=boolean
  Sum : Sum  Inputs=-+
  Sum2 : Sum  Inputs=-+|
  X-Axis Stiction Force : Fcn  Expr=-u(1) * (1+sgn(u(1))*u(2))
  stiction limit force : Gain  Gain=mu_stick
  F_Stick [N] : Outport  OutputWhenDisabled=reset  InitialOutput=0
      settings: AttributesFormatString=when disabled: %<OutputWhenDisabled>\ninitial: %<InitialOutput>
  Sliding! : Outport  Port=2  OutputWhenDisabled=reset  InitialOutput=0
      settings: AttributesFormatString=when disabled: %<OutputWhenDisabled>\ninitial: %<InitialOutput>
  wires:
  F_Normal [N]/1 -> stiction limit force/1, Positive1/1
  Sum2/1 -> Gain3/1  "dx"
  pos [m]/1 -> Sum2/2
  posFP [m]/1 -> Sum2/1
  vel [m/s]/1 -> Gain4/1
  Sum/1 -> Positive/1
  Memory/1 -> FixPt Relational Operator/2
  Positive/1 -> FixPt Relational Operator/1, Memory/1
  Abs./1 -> Sum/2
  Mux1/1 -> X-Axis Stiction Force/1
  Gain3/1 -> Mux1/1
  Gain4/1 -> Mux1/2
  FixPt Relational Operator/1 -> Sliding!/1
  Abs/1 -> Sum/1
  stiction limit force/1 -> Abs/1
  X-Axis Stiction Force/1 -> Check Vertical Friction/1
  Positive1/1 -> Check Vertical Friction/2
  Check Vertical Friction/1 -> F_Stick [N]/1, Abs./1

== system nmc_full_body_simmechanics_3fbl_2014a/Body Mechanics Layer (from Geyer s 2010 model)/Right Heel Contact/Ground Friction Model/Friction Switch ==
  note: Static/Kinetic Friction Switch
  Slide! : Inport
  Stick! : Inport  Port=2
  Memory : Memory
  S-R Flip-Flop : simulink_extras/Flip Flops/S-R Flip-Flop  initial_condition=1
  Terminator : Terminator
  Stiction : Outport
  wires:
  Memory/1 -> Stiction/1
  Slide!/1 -> S-R Flip-Flop/2
  Stick!/1 -> S-R Flip-Flop/1
  S-R Flip-Flop/2 -> Terminator/1
  S-R Flip-Flop/1 -> Memory/1

== system nmc_full_body_simmechanics_3fbl_2014a/Body Mechanics Layer (from Geyer s 2010 model)/Right Heel Contact/Ground Friction Model/X-Axis Kinetic Friction Model ==
  note: Sliding Limit Detector
  note: Footpoint Determiner
  note: Kinetic Friction Model
  pos [m] : Inport
  vel [m/s] : Inport  Port=2
  F_Normal [N] : Inport  Port=3
  Enable : EnablePort  StatesWhenEnabling=reset  ZeroCross=off
  Abs : Abs
  Constant : Constant  Value=vLimit
  FixPt Relational Operator : RelationalOperator  Operator=>  OutDataTypeStr=boolean  ZeroCross=off
  Memory : Memory
  Negative : simulink/Logic and Bit Operations/Compare To Zero  relop=<  OutDataTypeStr=boolean
  Product : Product  RndMeth=Zero
  Sign1 : Signum
  Sum : Sum  Inputs=|+-
  reverse : Gain  Gain=-1
  sliding friction coefficient : Gain  Gain=mu_slide
  posFP [m] : Outport  InitialOutput=0
      settings: AttributesFormatString=initial = '%<InitialOutput>'\nwhen disabled = '%<OutputWhenDisabled>'
  Stiction! : Outport  Port=2  OutputWhenDisabled=reset  InitialOutput=0
      settings: AttributesFormatString=initial = '%<InitialOutput>'\nwhen disabled = '%<OutputWhenDisabled>'
  F_Slide [N] : Outport  Port=3  OutputWhenDisabled=reset  InitialOutput=0
      settings: AttributesFormatString=initial = '%<InitialOutput>'\nwhen disabled = '%<OutputWhenDisabled>'
  wires:
  Constant/1 -> Sum/2
  Sum/1 -> Negative/1
  Abs/1 -> Sum/1
  Negative/1 -> Memory/1, FixPt Relational Operator/1
  Memory/1 -> FixPt Relational Operator/2
  FixPt Relational Operator/1 -> Stiction!/1
  Sign1/1 -> reverse/1
  sliding friction coefficient/1 -> Product/2
  Product/1 -> F_Slide [N]/1
  pos [m]/1 -> posFP [m]/1
  vel [m/s]/1 -> Abs/1, Sign1/1
  F_Normal [N]/1 -> sliding friction coefficient/1
  reverse/1 -> Product/1

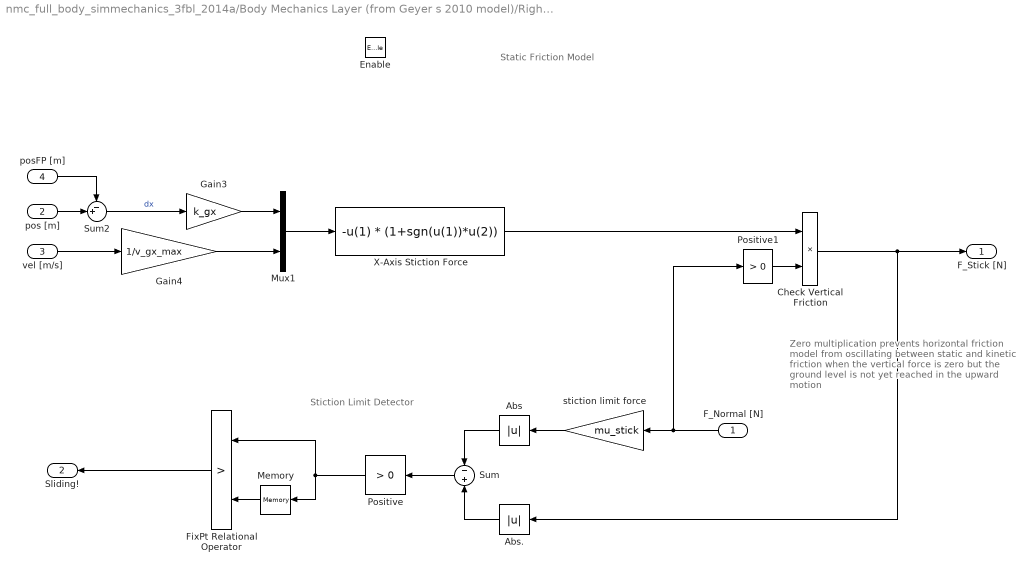
== system nmc_full_body_simmechanics_3fbl_2014a/Body Mechanics Layer (from Geyer s 2010 model)/Right Heel Contact/Ground Friction Model/X-Axis Static Friction Model ==
  note: Static Friction Model
  note: Stiction Limit Detector
  note: Zero multiplication prevents
      | horizontal friction model from
      | oscillating between static and kinetic
      | friction when the vertical force is zero but
      | the ground level is not yet reached
      | in the upward motion
  F_Normal [N] : Inport
  pos [m] : Inport  Port=2
  vel [m/s] : Inport  Port=3
  posFP [m] : Inport  Port=4
  Enable : EnablePort  StatesWhenEnabling=reset  ZeroCross=off
  Abs : Abs
  Abs. : Abs
  Check Vertical Friction : Product  RndMeth=Zero
  FixPt Relational Operator : RelationalOperator  Operator=>  OutDataTypeStr=boolean  ZeroCross=off
  Gain3 : Gain  Gain=k_gx
  Gain4 : Gain  Gain=1/v_gx_max
  Memory : Memory
  Mux1 : Mux  Inputs=2
  Positive : simulink/Logic and Bit Operations/Compare To Zero  relop=>  OutDataTypeStr=boolean
  Positive1 : simulink/Logic and Bit Operations/Compare To Zero  relop=>  OutDataTypeStr=boolean
  Sum : Sum  Inputs=-+
  Sum2 : Sum  Inputs=-+|
  X-Axis Stiction Force : Fcn  Expr=-u(1) * (1+sgn(u(1))*u(2))
  stiction limit force : Gain  Gain=mu_stick
  F_Stick [N] : Outport  OutputWhenDisabled=reset  InitialOutput=0
      settings: AttributesFormatString=when disabled: %<OutputWhenDisabled>\ninitial: %<InitialOutput>
  Sliding! : Outport  Port=2  OutputWhenDisabled=reset  InitialOutput=0
      settings: AttributesFormatString=when disabled: %<OutputWhenDisabled>\ninitial: %<InitialOutput>
  wires:
  F_Normal [N]/1 -> stiction limit force/1, Positive1/1
  Sum2/1 -> Gain3/1  "dx"
  pos [m]/1 -> Sum2/2
  posFP [m]/1 -> Sum2/1
  vel [m/s]/1 -> Gain4/1
  Sum/1 -> Positive/1
  Memory/1 -> FixPt Relational Operator/2
  Positive/1 -> FixPt Relational Operator/1, Memory/1
  Abs./1 -> Sum/2
  Mux1/1 -> X-Axis Stiction Force/1
  Gain3/1 -> Mux1/1
  Gain4/1 -> Mux1/2
  FixPt Relational Operator/1 -> Sliding!/1
  Abs/1 -> Sum/1
  stiction limit force/1 -> Abs/1
  X-Axis Stiction Force/1 -> Check Vertical Friction/1
  Positive1/1 -> Check Vertical Friction/2
  Check Vertical Friction/1 -> F_Stick [N]/1, Abs./1

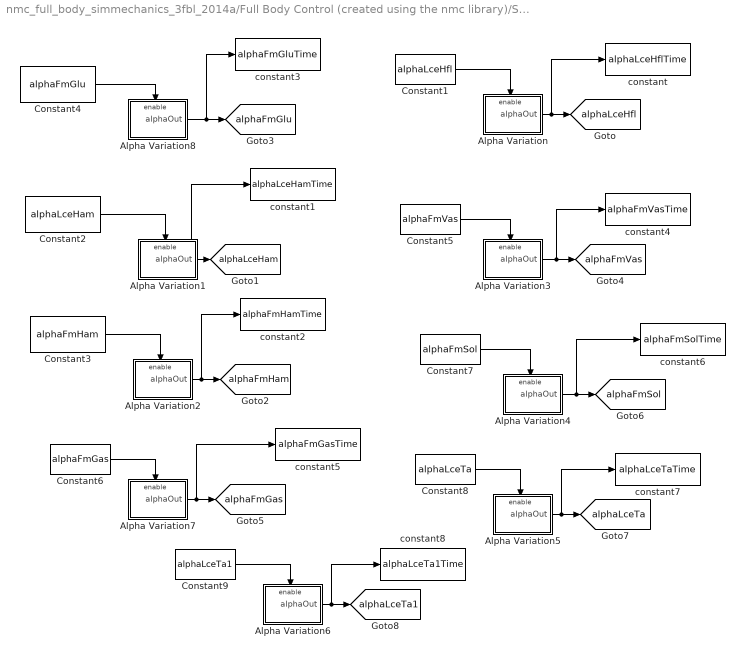
== system nmc_full_body_simmechanics_3fbl_2014a/Full Body Control (created using the nmc library)/Subsystem/Parameter variation/Alpha variation ==
  Alpha Variation : Subsystem
  Alpha Variation1 : Subsystem
  Alpha Variation2 : Subsystem
  Alpha Variation3 : Subsystem
  Alpha Variation4 : Subsystem
  Alpha Variation5 : Subsystem
  Alpha Variation6 : Subsystem
  Alpha Variation7 : Subsystem
  Alpha Variation8 : Subsystem
  Constant1 : Constant  Value=alphaLceHfl
  Constant2 : Constant  Value=alphaLceHam
  Constant3 : Constant  Value=alphaFmHam
  Constant4 : Constant  Value=alphaFmGlu
  Constant5 : Constant  Value=alphaFmVas
  Constant6 : Constant  Value=alphaFmGas
  Constant7 : Constant  Value=alphaFmSol
  Constant8 : Constant  Value=alphaLceTa
  Constant9 : Constant  Value=alphaLceTa1
  constant : ToWorkspace  VariableName=alphaLceHflTime  SaveFormat=Timeseries  SampleTime=-1
  constant1 : ToWorkspace  VariableName=alphaLceHamTime  SaveFormat=Timeseries  SampleTime=-1
  constant2 : ToWorkspace  VariableName=alphaFmHamTime  SaveFormat=Timeseries  SampleTime=-1
  constant3 : ToWorkspace  VariableName=alphaFmGluTime  SaveFormat=Timeseries  SampleTime=-1
  constant4 : ToWorkspace  VariableName=alphaFmVasTime  SaveFormat=Timeseries  SampleTime=-1
  constant5 : ToWorkspace  VariableName=alphaFmGasTime  SaveFormat=Timeseries  SampleTime=-1
  constant6 : ToWorkspace  VariableName=alphaFmSolTime  SaveFormat=Timeseries  SampleTime=-1
  constant7 : ToWorkspace  VariableName=alphaLceTaTime  SaveFormat=Timeseries  SampleTime=-1
  constant8 : ToWorkspace  VariableName=alphaLceTa1Time  SaveFormat=Timeseries  SampleTime=-1
  tag scope: alphaFmGas=global, alphaFmGlu=global, alphaFmHam=global, alphaFmSol=global, alphaFmVas=global, alphaLceHam=global, alphaLceHfl=global, alphaLceTa1=global, alphaLceTa=global
  wires:
  Alpha Variation/1("alphaOut ") -> constant/1, [alphaLceHfl]
  Alpha Variation1/1("alphaOut ") -> constant1/1, [alphaLceHam]
  Alpha Variation2/1("alphaOut ") -> [alphaFmHam], constant2/1
  Constant3/1 -> Alpha Variation2/Enable
  Constant4/1 -> Alpha Variation8/Enable
  Alpha Variation8/1("alphaOut ") -> constant3/1, [alphaFmGlu]
  Constant5/1 -> Alpha Variation3/Enable
  Alpha Variation6/1("alphaOut ") -> constant8/1, [alphaLceTa1]
  Alpha Variation3/1("alphaOut ") -> constant4/1, [alphaFmVas]
  Alpha Variation7/1("alphaOut ") -> constant5/1, [alphaFmGas]
  Constant6/1 -> Alpha Variation7/Enable
  Constant7/1 -> Alpha Variation4/Enable
  Alpha Variation4/1("alphaOut ") -> constant6/1, [alphaFmSol]
  Alpha Variation5/1("alphaOut ") -> constant7/1, [alphaLceTa]
  Constant8/1 -> Alpha Variation5/Enable
  Constant9/1 -> Alpha Variation6/Enable
  Constant2/1 -> Alpha Variation1/Enable
  Constant1/1 -> Alpha Variation/Enable

== system nmc_full_body_simmechanics_3fbl_2014a/Full Body Control (created using the nmc library)/Subsystem/Parameter variation/Amplitude Variation ==
  Add : Sum  Inputs=+++
  Constant1 : Constant  Value=amp_var
  Constant17 : Constant  Value=Amp
  Demux : Demux  Outputs=3
  Down : Subsystem
  "Off " : Subsystem
  Up : Subsystem
  constant10 : ToWorkspace  VariableName=ampTime  SaveFormat=Timeseries  SampleTime=-1
  tag scope: amp=global
  wires:
  Down/1("AmpDown ") -> Add/3
  Add/1 -> constant10/1, [amp]
  Demux/2 -> Up/Enable
  Demux/1 -> "Off "/Enable
  "Off "/1("Amp ") -> Add/1
  Constant1/1 -> Demux/1
  Demux/3 -> Down/Enable
  Up/1("AmpUp ") -> Add/2
  Constant17/1 -> Down/1(Amp), "Off "/1(Amp), Up/1(Amp)

== system nmc_full_body_simmechanics_3fbl_2014a/Full Body Control (created using the nmc library)/Subsystem/Parameter variation/Freq variation ==
  Add : Sum  Inputs=+++
  Constant1 : Constant  Value=freq_var
  Constant17 : Constant  Value=freq
  Demux : Demux  Outputs=3
  Down : Subsystem
  "Off " : Subsystem
  Up : Subsystem
  constant10 : ToWorkspace  VariableName=freqTime  SaveFormat=Timeseries  SampleTime=-1
  tag scope: freq=global
  wires:
  Down/1("freqDown ") -> Add/3
  Add/1 -> constant10/1, [freq]
  Demux/2 -> Up/Enable
  Demux/1 -> "Off "/Enable
  "Off "/1("Amp ") -> Add/1
  Constant1/1 -> Demux/1
  Demux/3 -> Down/Enable
  Up/1("freqUp ") -> Add/2
  Constant17/1 -> Down/1("freq "), "Off "/1(freq), Up/1("freq ")

== system nmc_full_body_simmechanics_3fbl_2014a/Full Body Control (created using the nmc library)/Subsystem/Parameter variation/Alpha variation/Alpha Variation ==
  alpha : EnablePort  ShowOutputPort=on
  Gain : Gain  Gain=10
  Gain1 : Gain  Gain=0.1
  Ramp : simulink/Sources/Ramp  slope=0.05  start=2  X0=0
  Rounding Function : Rounding  Operator=round
  Saturation : Saturate  UpperLimit=1  LowerLimit=0
  Switch : Switch  Threshold=1
  "alphaOut " : Outport
  wires:
  Switch/1 -> "alphaOut "/1
  Ramp/1 -> Gain/1
  alpha/1 -> Switch/2, Switch/3
  Saturation/1 -> Switch/1
  Gain/1 -> Rounding Function/1
  Rounding Function/1 -> Gain1/1
  Gain1/1 -> Saturation/1

== system nmc_full_body_simmechanics_3fbl_2014a/Full Body Control (created using the nmc library)/Subsystem/Parameter variation/Alpha variation/Alpha Variation1 ==
  alpha : EnablePort  ShowOutputPort=on
  Gain : Gain  Gain=10
  Gain1 : Gain  Gain=0.1
  Ramp : simulink/Sources/Ramp  slope=0.05  start=2  X0=0
  Rounding Function : Rounding  Operator=round
  Saturation : Saturate  UpperLimit=1  LowerLimit=0
  Switch : Switch  Threshold=1
  "alphaOut " : Outport
  wires:
  Switch/1 -> "alphaOut "/1
  Ramp/1 -> Gain/1
  alpha/1 -> Switch/2, Switch/3
  Saturation/1 -> Switch/1
  Gain/1 -> Rounding Function/1
  Rounding Function/1 -> Gain1/1
  Gain1/1 -> Saturation/1

== system nmc_full_body_simmechanics_3fbl_2014a/Full Body Control (created using the nmc library)/Subsystem/Parameter variation/Alpha variation/Alpha Variation2 ==
  alpha : EnablePort  ShowOutputPort=on
  Gain : Gain  Gain=10
  Gain1 : Gain  Gain=0.1
  Ramp : simulink/Sources/Ramp  slope=0.05  start=2  X0=0
  Rounding Function : Rounding  Operator=round
  Saturation : Saturate  UpperLimit=1  LowerLimit=0
  Switch : Switch  Threshold=1
  "alphaOut " : Outport
  wires:
  Switch/1 -> "alphaOut "/1
  Ramp/1 -> Gain/1
  alpha/1 -> Switch/2, Switch/3
  Saturation/1 -> Switch/1
  Gain/1 -> Rounding Function/1
  Rounding Function/1 -> Gain1/1
  Gain1/1 -> Saturation/1

== system nmc_full_body_simmechanics_3fbl_2014a/Full Body Control (created using the nmc library)/Subsystem/Parameter variation/Alpha variation/Alpha Variation3 ==
  alpha : EnablePort  ShowOutputPort=on
  Gain : Gain  Gain=10
  Gain1 : Gain  Gain=0.1
  Ramp : simulink/Sources/Ramp  slope=0.05  start=2  X0=0
  Rounding Function : Rounding  Operator=round
  Saturation : Saturate  UpperLimit=1  LowerLimit=0
  Switch : Switch  Threshold=1
  "alphaOut " : Outport
  wires:
  Switch/1 -> "alphaOut "/1
  Ramp/1 -> Gain/1
  alpha/1 -> Switch/2, Switch/3
  Saturation/1 -> Switch/1
  Gain/1 -> Rounding Function/1
  Rounding Function/1 -> Gain1/1
  Gain1/1 -> Saturation/1

== system nmc_full_body_simmechanics_3fbl_2014a/Full Body Control (created using the nmc library)/Subsystem/Parameter variation/Alpha variation/Alpha Variation4 ==
  alpha : EnablePort  ShowOutputPort=on
  Gain : Gain  Gain=10
  Gain1 : Gain  Gain=0.1
  Ramp : simulink/Sources/Ramp  slope=0.05  start=2  X0=0
  Rounding Function : Rounding  Operator=round
  Saturation : Saturate  UpperLimit=1  LowerLimit=0
  Switch : Switch  Threshold=1
  "alphaOut " : Outport
  wires:
  Switch/1 -> "alphaOut "/1
  Ramp/1 -> Gain/1
  alpha/1 -> Switch/2, Switch/3
  Saturation/1 -> Switch/1
  Gain/1 -> Rounding Function/1
  Rounding Function/1 -> Gain1/1
  Gain1/1 -> Saturation/1

== system nmc_full_body_simmechanics_3fbl_2014a/Full Body Control (created using the nmc library)/Subsystem/Parameter variation/Alpha variation/Alpha Variation5 ==
  alpha : EnablePort  ShowOutputPort=on
  Gain : Gain  Gain=10
  Gain1 : Gain  Gain=0.1
  Ramp : simulink/Sources/Ramp  slope=0.05  start=2  X0=0
  Rounding Function : Rounding  Operator=round
  Saturation : Saturate  UpperLimit=1  LowerLimit=0
  Switch : Switch  Threshold=1
  "alphaOut " : Outport
  wires:
  Switch/1 -> "alphaOut "/1
  Ramp/1 -> Gain/1
  alpha/1 -> Switch/2, Switch/3
  Saturation/1 -> Switch/1
  Gain/1 -> Rounding Function/1
  Rounding Function/1 -> Gain1/1
  Gain1/1 -> Saturation/1

== system nmc_full_body_simmechanics_3fbl_2014a/Full Body Control (created using the nmc library)/Subsystem/Parameter variation/Alpha variation/Alpha Variation6 ==
  alpha : EnablePort  ShowOutputPort=on
  Gain : Gain  Gain=10
  Gain1 : Gain  Gain=0.1
  Ramp : simulink/Sources/Ramp  slope=0.05  start=2  X0=0
  Rounding Function : Rounding  Operator=round
  Saturation : Saturate  UpperLimit=1  LowerLimit=0
  Switch : Switch  Threshold=1
  "alphaOut " : Outport
  wires:
  Switch/1 -> "alphaOut "/1
  Ramp/1 -> Gain/1
  alpha/1 -> Switch/2, Switch/3
  Saturation/1 -> Switch/1
  Gain/1 -> Rounding Function/1
  Rounding Function/1 -> Gain1/1
  Gain1/1 -> Saturation/1

== system nmc_full_body_simmechanics_3fbl_2014a/Full Body Control (created using the nmc library)/Subsystem/Parameter variation/Alpha variation/Alpha Variation7 ==
  alpha : EnablePort  ShowOutputPort=on
  Gain : Gain  Gain=10
  Gain1 : Gain  Gain=0.1
  Ramp : simulink/Sources/Ramp  slope=0.05  start=2  X0=0
  Rounding Function : Rounding  Operator=round
  Saturation : Saturate  UpperLimit=1  LowerLimit=0
  Switch : Switch  Threshold=1
  "alphaOut " : Outport
  wires:
  Switch/1 -> "alphaOut "/1
  Ramp/1 -> Gain/1
  alpha/1 -> Switch/2, Switch/3
  Saturation/1 -> Switch/1
  Gain/1 -> Rounding Function/1
  Rounding Function/1 -> Gain1/1
  Gain1/1 -> Saturation/1

== system nmc_full_body_simmechanics_3fbl_2014a/Full Body Control (created using the nmc library)/Subsystem/Parameter variation/Alpha variation/Alpha Variation8 ==
  alpha : EnablePort  ShowOutputPort=on
  Gain : Gain  Gain=10
  Gain1 : Gain  Gain=0.1
  Ramp : simulink/Sources/Ramp  slope=0.05  start=2  X0=0
  Rounding Function : Rounding  Operator=round
  Saturation : Saturate  UpperLimit=1  LowerLimit=0
  Switch : Switch  Threshold=1
  "alphaOut " : Outport
  wires:
  Switch/1 -> "alphaOut "/1
  Ramp/1 -> Gain/1
  alpha/1 -> Switch/2, Switch/3
  Saturation/1 -> Switch/1
  Gain/1 -> Rounding Function/1
  Rounding Function/1 -> Gain1/1
  Gain1/1 -> Saturation/1

== system nmc_full_body_simmechanics_3fbl_2014a/Full Body Control (created using the nmc library)/Subsystem/Parameter variation/Amplitude Variation/Down ==
  Amp : Inport
  Enable : EnablePort
  Gain : Gain  Gain=10
  Gain1 : Gain  Gain=0.1
  Ramp : simulink/Sources/Ramp  slope=0.04  start=2  X0=0
  Rounding Function : Rounding  Operator=round
  Saturation : Saturate  UpperLimit=1.5  LowerLimit=0
  Subtract : Sum  Inputs=+-
  "AmpDown " : Outport
  wires:
  Saturation/1 -> Subtract/2
  Ramp/1 -> Gain/1
  Amp/1 -> Subtract/1
  Gain/1 -> Rounding Function/1
  Rounding Function/1 -> Gain1/1
  Gain1/1 -> Saturation/1
  Subtract/1 -> "AmpDown "/1

== system nmc_full_body_simmechanics_3fbl_2014a/Full Body Control (created using the nmc library)/Subsystem/Parameter variation/Amplitude Variation/Off  ==
  Amp : Inport
  Enable : EnablePort
  "Amp " : Outport
  wires:
  Amp/1 -> "Amp "/1
